simulink model "g_errors"  (R2023b)
settings: Solver=VariableStepAuto  StartTime=0.0  StopTime=0.1  RelTol=1e-3
libraries: sensors_subsystems x1
settings Model: Creator=brent  LastModifiedBy=brent

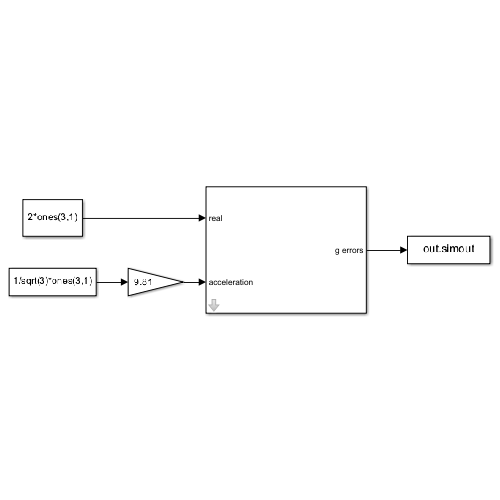
[thumbnail: Simulink's stored preview of the top-level diagram]
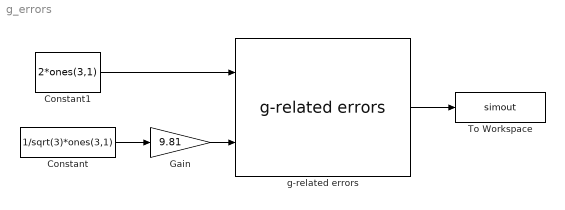
== system g_errors ==
  Constant : Constant  Value=1/sqrt(3)*ones(3,1)
  Constant1 : Constant  Value=2*ones(3,1)
  Gain : Gain  Gain=9.81
  To Workspace : ToWorkspace  VariableName=simout  SampleTime=-1
      settings: Save2DSignal=2-D array (concatenate along first dimension)
  g-related errors : sensors_subsystems/g-related errors  gyro=gyro
      settings: SourceProductName=Sensors library
  wires:
  Constant/1 -> Gain/1
  Gain/1 -> g-related errors/2
  Constant1/1 -> g-related errors/1
  g-related errors/1 -> To Workspace/1
